simulink model "StandaloneDAQv07_R2014a"  (R2014a)
settings: Solver=FixedStepDiscrete  SolverMode=MultiTasking  StartTime=0.0  StopTime=inf  FixedStep=0.0005  RelTol=1e-3
values from neighbouring files (symbols this model uses):
  ANOMALY_INIT = 10    [DAQParams3_1ms_DDA.m]
  Calibration = getCalibrationParams_ATRIAS()    [DAQParams3_1ms_DDA.m]
  EnableFT = 0    [DAQParams3_1ms_DDA.m]
  EncoderAngleLimits = [60 240; 120 300; 60 240; 120 300; 60 240; 120 300; 60 240; 120 300; -30 30; -30 30; -inf inf; -inf inf; -inf inf; -inf inf; -30 30; -30 30; -inf inf; -90 90; -90 90]*pi/180    [DAQParams3_1ms_DDA.m]
  EncoderFiltSys = getDerivFilter(2, 5, 5, Ts)    [DAQParams3_1ms_DDA.m]
  EncoderThreshold = [5; 5; 5; 5; 5; 5; 5; 5; 5; 5; 250; 250; 250; 250; 5; 5; 5; 5; 5]*pi/180    [DAQParams3_1ms_DDA.m]
  IMUAngleLimits = [-180 180; -90 90; -90 90]*pi/180    [DAQParams3_1ms_DDA.m]
  IMUCommand = 70    [DAQParams3_1ms_DDA.m]
  IMUThreshold = 5*pi/180    (= 0.0872664625997)    [DAQParams3_1ms_DDA.m]
  MAX_ANOMALY = 30    [DAQParams3_1ms_DDA.m]
  MedullaCommand = 0    [DAQParams3_1ms_DDA.m]
  MicrostrainFiltSys = getDerivFilter(2, 5, 5, TsMicrostrain)    [DAQParams3_1ms_DDA.m]
  MODBUS_TIMEOUT = 0.02    [DAQParams3_1ms_DDA.m]
  ResetDAQ = 0    [DAQParams3_1ms_DDA.m]
  ResetYaw = 0    [DAQParams3_1ms_DDA.m]
  STREAMING_TIMEOUT = 0.1    [DAQParams3_1ms_DDA.m]
  TareFT = 0    [DAQParams3_1ms_DDA.m]
  Ts = 0.001    [DAQParams3_1ms_DDA.m]
  UseMicrostrainRate = 0    [DAQParams3_1ms_DDA.m]
undefined symbols (not defined in the file or in its folder): FTCalibration, GearOffset, IMUTorsoOffset, m_XR17D15x, standard
libraries: xpcethercatlib x167, speedgoatlib x13, dspswit3 x2, simulink x2, xpcseriallib x1, SpeedgoatModified x1
(part 1 of 4)
settings Model: xpc_rtwmakecfg_data=_xpcethercatlib_  ParamWorkspaceSource=ReferencedWorkspace  TunableVars=EnableFT,GearOffset,IMUCommand,IMUTorsoOffset,MedullaCommand,ResetDAQ,ResetYaw,TareFT  TunableVarsStorageClass=Auto,Auto,Auto,Auto,Auto,Auto,Auto,Auto  TunableVarsTypeQualifier=,,,,,,,  ExplicitPartitioning=on  Creator=bgbuss  LastModifiedBy=bgbuss
settings SolverCC: EnableConcurrentExecution=on
settings DataIOCC: LimitDataPoints=off
settings OptimizationCC: InlineParams=on  ExpressionDepthLimit=2147483647
settings DebuggingCC: UniqueDataStoreMsg=error  StateNameClashWarn=warning
settings HardwareCC: ProdIntDivRoundTo=Zero  ProdEndianess=LittleEndian  ProdHWDeviceType=Generic->32-bit x86 compatible
settings SFSimCC: SimUserIncludeDirs=./DynamicModel/c
settings RTWCC: SystemTargetFile=slrt.tlc  TLCOptions=-axPCModelStackSizeKB=128 -axPCMaxOverloads=100  TemplateMakefile=slrt_default_tmf  Description=Simulink Real-Time  ProcessScript=slrt_make_rtw_hook  RTWUseSimCustomCode=on  CustomInclude=./DynamicModel/c  CodeExecutionProfiling=on  CodeProfilingSaveOptions=AllData  RTWCompilerOptimization=On
settings CodeAppCC: MATLABSourceComments=on
settings SimulinkRealTimeCC: GeneratePreprocessorConditionals=Disable all  EnableShiftOperators=on  RL32LogBufSizeModifier=100000000  xPCTaskExecutionProfile=on  xPCRL32EventNumber=250000  xPCisModelTimeout=off  xPCModelTimeoutSecs=20

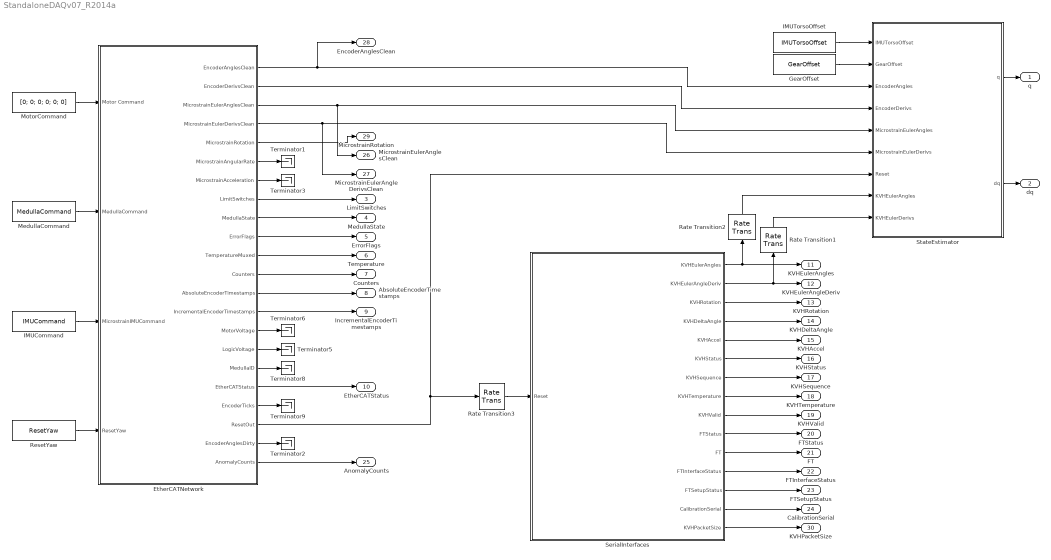
== system StandaloneDAQv07_R2014a ==
  EtherCATNetwork : Subsystem
  GearOffset : Constant  Value=GearOffset
  IMUCommand : Constant  Value=IMUCommand
  IMUTorsoOffset : Constant  Value=IMUTorsoOffset
  MedullaCommand : Constant  Value=MedullaCommand
  MotorCommand : Constant  Value=[0; 0; 0; 0; 0; 0]
  Rate Transition1 : RateTransition  OutPortSampleTime=Ts
  Rate Transition2 : RateTransition  OutPortSampleTime=Ts
  Rate Transition3 : RateTransition  OutPortSampleTime=0.001
  ResetYaw : Constant  Value=ResetYaw  OutDataTypeStr=boolean
  SerialInterfaces : Subsystem  TreatAsAtomicUnit=on  SystemSampleTime=0.001
  StateEstimator : Subsystem
  Terminator{1..3,5..6,8..9} (7 alike) : Terminator
  q : Outport
  dq : Outport  Port=2
  LimitSwitches : Outport  Port=3
  MedullaState : Outport  Port=4
  ErrorFlags : Outport  Port=5
  Temperature : Outport  Port=6
  Counters : Outport  Port=7
  AbsoluteEncoderTimestamps : Outport  Port=8
  IncrementalEncoderTimestamps : Outport  Port=9
  EtherCATStatus : Outport  Port=10
  KVHEulerAngles : Outport  Port=11
  KVHEulerAngleDeriv : Outport  Port=12
  KVHRotation : Outport  Port=13
  KVHDeltaAngle : Outport  Port=14
  KVHAccel : Outport  Port=15
  KVHStatus : Outport  Port=16
  KVHSequence : Outport  Port=17
  KVHTemperature : Outport  Port=18
  KVHValid : Outport  Port=19
  FTStatus : Outport  Port=20
  FT : Outport  Port=21
  FTInterfaceStatus : Outport  Port=22
  FTSetupStatus : Outport  Port=23
  CalibrationSerial : Outport  Port=24
  AnomalyCounts : Outport  Port=25
  MicrostrainEulerAnglesClean : Outport  Port=26
  MicrostrainEulerAngleDerivsClean : Outport  Port=27
  EncoderAnglesClean : Outport  Port=28
  MicrostrainRotation : Outport  Port=29
  KVHPacketSize : Outport  Port=30
  wires:
  EtherCATNetwork/8(LimitSwitches) -> LimitSwitches/1
  EtherCATNetwork/10(ErrorFlags) -> ErrorFlags/1
  EtherCATNetwork/15(MotorVoltage) -> Terminator6/1
  EtherCATNetwork/5(MicrostrainRotation) -> MicrostrainRotation/1
  EtherCATNetwork/9(MedullaState) -> MedullaState/1
  EtherCATNetwork/16(LogicVoltage) -> Terminator5/1
  EtherCATNetwork/11(TemperatureMuxed) -> Temperature/1
  EtherCATNetwork/18(EtherCATStatus) -> EtherCATStatus/1
  EtherCATNetwork/12(Counters) -> Counters/1
  StateEstimator/1(q) -> q/1
  StateEstimator/2(dq) -> dq/1
  EtherCATNetwork/22(AnomalyCounts) -> AnomalyCounts/1
  MotorCommand/1 -> EtherCATNetwork/1(Motor Command)
  MedullaCommand/1 -> EtherCATNetwork/2(MedullaCommand)
  IMUCommand/1 -> EtherCATNetwork/3(MicrostrainIMUCommand)
  EtherCATNetwork/17(MedullaID) -> Terminator8/1
  EtherCATNetwork/19(EncoderTicks) -> Terminator9/1
  EtherCATNetwork/7(MicrostrainAcceleration) -> Terminator3/1
  EtherCATNetwork/13(AbsoluteEncoderTimestamps) -> AbsoluteEncoderTimestamps/1
  EtherCATNetwork/14(IncrementalEncoderTimestamps) -> IncrementalEncoderTimestamps/1
  SerialInterfaces/10(FTStatus) -> FTStatus/1
  SerialInterfaces/11(FT) -> FT/1
  SerialInterfaces/12(FTInterfaceStatus) -> FTInterfaceStatus/1
  SerialInterfaces/13(FTSetupStatus) -> FTSetupStatus/1
  SerialInterfaces/14(CalibrationSerial) -> CalibrationSerial/1
  SerialInterfaces/3(KVHRotation) -> KVHRotation/1
  SerialInterfaces/2(KVHEulerAngleDeriv) -> KVHEulerAngleDeriv/1, Rate Transition1/1
  SerialInterfaces/1(KVHEulerAngles) -> Rate Transition2/1, KVHEulerAngles/1
  SerialInterfaces/7(KVHSequence) -> KVHSequence/1
  SerialInterfaces/8(KVHTemperature) -> KVHTemperature/1
  SerialInterfaces/5(KVHAccel) -> KVHAccel/1
  SerialInterfaces/9(KVHValid) -> KVHValid/1
  SerialInterfaces/6(KVHStatus) -> KVHStatus/1
  SerialInterfaces/4(KVHDeltaAngle) -> KVHDeltaAngle/1
  IMUTorsoOffset/1 -> StateEstimator/1(IMUTorsoOffset)
  GearOffset/1 -> StateEstimator/2(GearOffset)
  Rate Transition2/1 -> StateEstimator/8(KVHEulerAngles)
  EtherCATNetwork/20(ResetOut) -> StateEstimator/7(Reset), Rate Transition3/1
  EtherCATNetwork/1(EncoderAnglesClean) -> EncoderAnglesClean/1, StateEstimator/3(EncoderAngles)
  EtherCATNetwork/3(MicrostrainEulerAnglesClean) -> StateEstimator/5(MicrostrainEulerAngles), MicrostrainEulerAnglesClean/1
  EtherCATNetwork/4(MicrostrainEulerDerivsClean) -> StateEstimator/6(" MicrostrainEulerDerivs"), MicrostrainEulerAngleDerivsClean/1
  Rate Transition3/1 -> SerialInterfaces/1(Reset)
  EtherCATNetwork/2(EncoderDerivsClean) -> StateEstimator/4(EncoderDerivs)
  Rate Transition1/1 -> StateEstimator/9(KVHEulerDerivs)
  EtherCATNetwork/6(MicrostrainAngularRate) -> Terminator1/1
  EtherCATNetwork/21(EncoderAnglesDirty) -> Terminator2/1
  ResetYaw/1 -> EtherCATNetwork/4(ResetYaw)
  SerialInterfaces/15(KVHPacketSize) -> KVHPacketSize/1

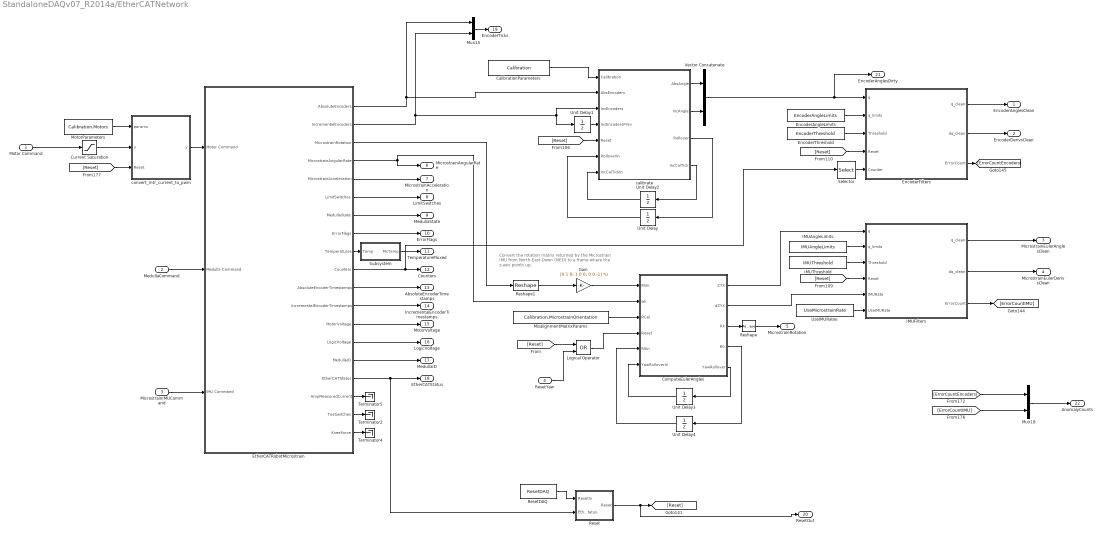
== system StandaloneDAQv07_R2014a/EtherCATNetwork ==
  note: Convert the rotation matrix returned by the
      | Microstrain IMU from North-East-Down
      | (NED) to a frame where the z-axis points up.
  Motor Command : Inport
  MedullaCommand : Inport  Port=2
  MicrostrainIMUCommand : Inport  Port=3
  ResetYaw : Inport  Port=4
  CalibrationParameters : Constant  Value=Calibration  OutDataTypeStr=Bus: RobotCalibrationBus
  ComputeEulerAngles : MATLAB Function  TreatAsAtomicUnit=on
  Current Saturation : Saturate  UpperLimit=50  LowerLimit=-50
  EncoderAngleLimits : Constant  Value=EncoderAngleLimits
  EncoderFilters : Subsystem  TreatAsAtomicUnit=on
  EncoderThreshold : Constant  Value=EncoderThreshold
  EtherCATRobotMicrostrain : Subsystem
  Gain : Gain  Gain=[0 1 0; 1 0 0; 0 0 -1]  Multiplication=Matrix(K*u)
  IMUAngleLimits : Constant  Value=IMUAngleLimits
  IMUFilters : Subsystem  TreatAsAtomicUnit=on
  IMUThreshold : Constant  Value=IMUThreshold
  Logical Operator : Logic  Operator=OR  OutDataTypeStr=boolean
  MisalignmentMatrixParams : Constant  Value=Calibration.MicrostrainOrientation
  MotorParameters : Constant  Value=Calibration.Motors
  Mux15 : Mux  Inputs=2
  Mux18 : Mux  Inputs=2
  Reset : Subsystem
  ResetDAQ : Constant  Value=ResetDAQ  OutDataTypeStr=boolean
  Reshape : Reshape
  Reshape1 : Reshape  OutputDimensionality=Customize  OutputDimensions=[3,3]
  Selector : Selector  IndexMode=Zero-based  InputPortWidth=7  Indices=[0 1 3 4 0 1 3 4 2 5 0 1 3 4 2 5 6 6 6]
  Subsystem : Subsystem
  Terminator2 : Terminator
  Terminator4 : Terminator
  Terminator5 : Terminator
  Unit Delay : UnitDelay  InitialCondition=zeros(9,1)  SampleTime=-1
  Unit Delay1 : UnitDelay  SampleTime=-1
  Unit Delay2 : UnitDelay  InitialCondition=zeros(6,1)  SampleTime=-1
  Unit Delay3 : UnitDelay  InitialCondition=[0; 0]  SampleTime=-1
  Unit Delay4 : UnitDelay  InitialCondition=zeros(3,3)  SampleTime=-1
  UseIMURates : Constant  Value=UseMicrostrainRate
  Vector Concatenate : Concatenate
  calibrate : MATLAB Function  TreatAsAtomicUnit=on
  convert_mtr_current_to_pwm : MATLAB Function  TreatAsAtomicUnit=on
  EncoderAnglesClean : Outport
  EncoderDerivsClean : Outport  Port=2
  MicrostrainEulerAnglesClean : Outport  Port=3
  MicrostrainEulerDerivsClean : Outport  Port=4
  MicrostrainRotation : Outport  Port=5
  MicrostrainAngularRate : Outport  Port=6
  MicrostrainAcceleration : Outport  Port=7
  LimitSwitches : Outport  Port=8
  MedullaState : Outport  Port=9
  ErrorFlags : Outport  Port=10
  TemperatureMuxed : Outport  Port=11
  Counters : Outport  Port=12
  AbsoluteEncoderTimestamps : Outport  Port=13
  IncrementalEncoderTimestamps : Outport  Port=14
  MotorVoltage : Outport  Port=15
  LogicVoltage : Outport  Port=16
  MedullaID : Outport  Port=17
  EtherCATStatus : Outport  Port=18
  EncoderTicks : Outport  Port=19
  ResetOut : Outport  Port=20
  EncoderAnglesDirty : Outport  Port=21
  AnomalyCounts : Outport  Port=22
  wires:
  EtherCATRobotMicrostrain/18(ToeSwitches) -> Terminator2/1
  EtherCATRobotMicrostrain/17(AmpMeasuredCurrent) -> Terminator5/1
  MicrostrainIMUCommand/1 -> EtherCATRobotMicrostrain/3(IMU Command)
  MedullaCommand/1 -> EtherCATRobotMicrostrain/2(Medulla Command)
  EtherCATRobotMicrostrain/16(EtherCATStatus) -> EtherCATStatus/1, Reset/2(EtherCATStatus)
  CalibrationParameters/1 -> calibrate/1(Calibration)
  calibrate/3(Rollover) -> Unit Delay/1
  Unit Delay/1 -> calibrate/6(RolloverIn)
  [Reset] -> calibrate/5(Reset)
  Reset/1(Reset) -> ResetOut/1, [Reset]
  ResetDAQ/1 -> Reset/1(ResetIn)
  Unit Delay1/1 -> calibrate/4(IncEncodersPrev)
  Unit Delay2/1 -> calibrate/7(IncCalTickIn)
  calibrate/4(IncCalTick) -> Unit Delay2/1
  [Reset] -> convert_mtr_current_to_pwm/3(Reset)
  Motor Command/1 -> Current Saturation/1
  MotorParameters/1 -> convert_mtr_current_to_pwm/1(params)
  Current Saturation/1 -> convert_mtr_current_to_pwm/2(u)
  convert_mtr_current_to_pwm/1(y) -> EtherCATRobotMicrostrain/1(Motor Command)
  Mux15/1 -> EncoderTicks/1
  EtherCATRobotMicrostrain/19(KneeForce) -> Terminator4/1
  EtherCATRobotMicrostrain/7(MedullaState) -> MedullaState/1
  Subsystem/1(MxTemp) -> TemperatureMuxed/1
  EtherCATRobotMicrostrain/9(Temperatures) -> Subsystem/1(Temp)
  EtherCATRobotMicrostrain/8(ErrorFlags) -> ErrorFlags/1
  EtherCATRobotMicrostrain/6(LimitSwitches) -> LimitSwitches/1
  EtherCATRobotMicrostrain/13(MotorVoltage) -> MotorVoltage/1
  EtherCATRobotMicrostrain/14(LogicVoltage) -> LogicVoltage/1
  EtherCATRobotMicrostrain/5(MicrostrainAcceleration) -> MicrostrainAcceleration/1
  EtherCATRobotMicrostrain/11(AbsoluteEncoderTimestamps) -> AbsoluteEncoderTimestamps/1
  EtherCATRobotMicrostrain/12(IncrementalEncoderTimestamps) -> IncrementalEncoderTimestamps/1
  EtherCATRobotMicrostrain/15(MedullaID) -> MedullaID/1
  EtherCATRobotMicrostrain/1(AbsoluteEncoders) -> Mux15/1, calibrate/2(AbsEncoders)
  EtherCATRobotMicrostrain/2(IncrementalEncoders) -> Mux15/2, calibrate/3(IncEncoders), Unit Delay1/1
  ComputeEulerAngles/1(ZYX) -> IMUFilters/1(q)
  [Reset] -> IMUFilters/4(Reset)
  IMUFilters/3(ErrorCount) -> [ErrorCountIMU]
  IMUThreshold/1 -> IMUFilters/3(Threshold)
  EtherCATRobotMicrostrain/10(Counters) -> Selector/1, Counters/1
  IMUAngleLimits/1 -> IMUFilters/2(q_limits)
  Selector/1 -> EncoderFilters/5(Counter)
  UseIMURates/1 -> IMUFilters/6(UseIMURate)
  EncoderFilters/3(ErrorCount) -> [ErrorCountEncoders]
  IMUFilters/2(dq_clean) -> MicrostrainEulerDerivsClean/1
  [Reset] -> EncoderFilters/4(Reset)
  EncoderAngleLimits/1 -> EncoderFilters/2(q_limits)
  EncoderFilters/1(q_clean) -> EncoderAnglesClean/1
  IMUFilters/1(q_clean) -> MicrostrainEulerAnglesClean/1
  EncoderFilters/2(dq_clean) -> EncoderDerivsClean/1
  EncoderThreshold/1 -> EncoderFilters/3(Threshold)
  calibrate/1(AbsAngle) -> Vector Concatenate/1
  calibrate/2(IncAngle) -> Vector Concatenate/2
  Vector Concatenate/1 -> EncoderAnglesDirty/1, EncoderFilters/1(q)
  ComputeEulerAngles/2(dZYX) -> IMUFilters/5(IMURate)
  Mux18/1 -> AnomalyCounts/1
  [ErrorCountEncoders] -> Mux18/1
  [ErrorCountIMU] -> Mux18/2
  MisalignmentMatrixParams/1 -> ComputeEulerAngles/3(RCal)
  Unit Delay4/1 -> ComputeEulerAngles/5(R0In)
  ComputeEulerAngles/4(R0) -> Unit Delay4/1
  ComputeEulerAngles/3(Rk) -> Reshape/1
  [Reset] -> Logical Operator/1
  Reshape/1 -> MicrostrainRotation/1
  EtherCATRobotMicrostrain/3(MicrostrainRotation) -> Reshape1/1
  EtherCATRobotMicrostrain/4(MicrostrainAngularRate) -> ComputeEulerAngles/2(wk), MicrostrainAngularRate/1
  ComputeEulerAngles/5(YawRollover) -> Unit Delay3/1
  Unit Delay3/1 -> ComputeEulerAngles/6(YawRolloverIn)
  ResetYaw/1 -> Logical Operator/2
  Logical Operator/1 -> ComputeEulerAngles/4(Reset)
  Reshape1/1 -> Gain/1
  Gain/1 -> ComputeEulerAngles/1(RkIn)

== system StandaloneDAQv07_R2014a/SerialInterfaces ==
  Reset : Inport
  EnableFT : Constant  Value=EnableFT  OutDataTypeStr=boolean
  FTInterface : Subsystem
  KVH : Subsystem
  ResetYaw : Constant  Value=ResetYaw  OutDataTypeStr=boolean
  TareFT : Constant  Value=TareFT  OutDataTypeStr=boolean
  KVHEulerAngles : Outport
  KVHEulerAngleDeriv : Outport  Port=2
  KVHRotation : Outport  Port=3
  KVHDeltaAngle : Outport  Port=4
  KVHAccel : Outport  Port=5
  KVHStatus : Outport  Port=6
  KVHSequence : Outport  Port=7
  KVHTemperature : Outport  Port=8
  KVHValid : Outport  Port=9
  FTStatus : Outport  Port=10
  FT : Outport  Port=11
  FTInterfaceStatus : Outport  Port=12
  FTSetupStatus : Outport  Port=13
  CalibrationSerial : Outport  Port=14
  KVHPacketSize : Outport  Port=15
  wires:
  KVH/4(DeltaAngle) -> KVHDeltaAngle/1
  KVH/5(Accel) -> KVHAccel/1
  KVH/7(Sequence) -> KVHSequence/1
  KVH/6(Status) -> KVHStatus/1
  KVH/8(Temperature) -> KVHTemperature/1
  KVH/9(Valid) -> KVHValid/1
  ResetYaw/1 -> KVH/1(ResetYaw)
  KVH/1(EulerAngles) -> KVHEulerAngles/1
  KVH/2(EulerAngleDerivatives) -> KVHEulerAngleDeriv/1
  FTInterface/4(FTSetupStatus) -> FTSetupStatus/1
  FTInterface/1(FTStatus) -> FTStatus/1
  FTInterface/5(CalibrationSerial) -> CalibrationSerial/1
  FTInterface/3(FTInterfaceStatus) -> FTInterfaceStatus/1
  TareFT/1 -> FTInterface/1(Tare)
  Reset/1 -> FTInterface/2(Reset), KVH/2(Reset)
  FTInterface/2(FT) -> FT/1
  KVH/3(Rk) -> KVHRotation/1
  EnableFT/1 -> FTInterface/Enable
  KVH/10(PacketSize) -> KVHPacketSize/1

== system StandaloneDAQv07_R2014a/StateEstimator ==
  IMUTorsoOffset : Inport
  GearOffset : Inport  Port=2
  EncoderAngles : Inport  Port=3
  EncoderDerivs : Inport  Port=4
  MicrostrainEulerAngles : Inport  Port=5
  " MicrostrainEulerDerivs" : Inport  Port=6
  Reset : Inport  Port=7
  KVHEulerAngles : Inport  Port=8
  KVHEulerDerivs : Inport  Port=9
  GeneralizedCoordinates : MATLAB Function  TreatAsAtomicUnit=on
  Switch : Switch  Criteria=u2 > Threshold
  Switch1 : Switch  Criteria=u2 > Threshold
  UseIMU : Constant
  UseKVH : Constant
  UseMotorIncEncoders : Constant
  q : Outport
  dq : Outport  Port=2
  wires:
  UseIMU/1 -> GeneralizedCoordinates/6(UseIMU)
  GearOffset/1 -> GeneralizedCoordinates/8(GearOffset)
  UseMotorIncEncoders/1 -> GeneralizedCoordinates/5(UseMotorIncEncoders)
  IMUTorsoOffset/1 -> GeneralizedCoordinates/7(IMUTorsoOffset)
  GeneralizedCoordinates/2(dq_clean) -> dq/1
  GeneralizedCoordinates/1(q_clean) -> q/1
  Reset/1 -> GeneralizedCoordinates/9(Reset)
  EncoderAngles/1 -> GeneralizedCoordinates/1(EncoderAngles)
  EncoderDerivs/1 -> GeneralizedCoordinates/2(EncoderVelocities)
  KVHEulerAngles/1 -> Switch/1
  MicrostrainEulerAngles/1 -> Switch/3
  Switch/1 -> GeneralizedCoordinates/3(IMUAngles)
  UseKVH/1 -> Switch1/2, Switch/2
  KVHEulerDerivs/1 -> Switch1/1
  " MicrostrainEulerDerivs"/1 -> Switch1/3
  Switch1/1 -> GeneralizedCoordinates/4(IMUVelocities)

== system StandaloneDAQv07_R2014a/EtherCATNetwork/EncoderFilters ==
  q : Inport  Partition=on  PartitionDimension=1  PartitionWidth=1
  q_limits : Inport  Port=2  Partition=on  PartitionDimension=1  PartitionWidth=1
  Threshold : Inport  Port=3  Partition=on  PartitionDimension=1  PartitionWidth=1
  Reset : Inport  Port=4  Partition=off
  Counter : Inport  Port=5  Partition=on  PartitionDimension=1  PartitionWidth=1
  CheckAndFilterEncoder : Subsystem
  For Each : ForEach  DisableCoverage=on  IndexMode=One-based
  q_clean : Outport  ConcatenationDimension=1
  dq_clean : Outport  Port=2  ConcatenationDimension=1
  ErrorCount : Outport  Port=3  ConcatenationDimension=1
  wires:
  Counter/1 -> CheckAndFilterEncoder/5(Counter)
  Reset/1 -> CheckAndFilterEncoder/4(Reset)
  CheckAndFilterEncoder/2(dq_clean) -> dq_clean/1
  q_limits/1 -> CheckAndFilterEncoder/2(q_limits)
  CheckAndFilterEncoder/3(ErrorCount) -> ErrorCount/1
  CheckAndFilterEncoder/1(q_clean) -> q_clean/1
  Threshold/1 -> CheckAndFilterEncoder/3(Threshold)
  q/1 -> CheckAndFilterEncoder/1(q_daq)

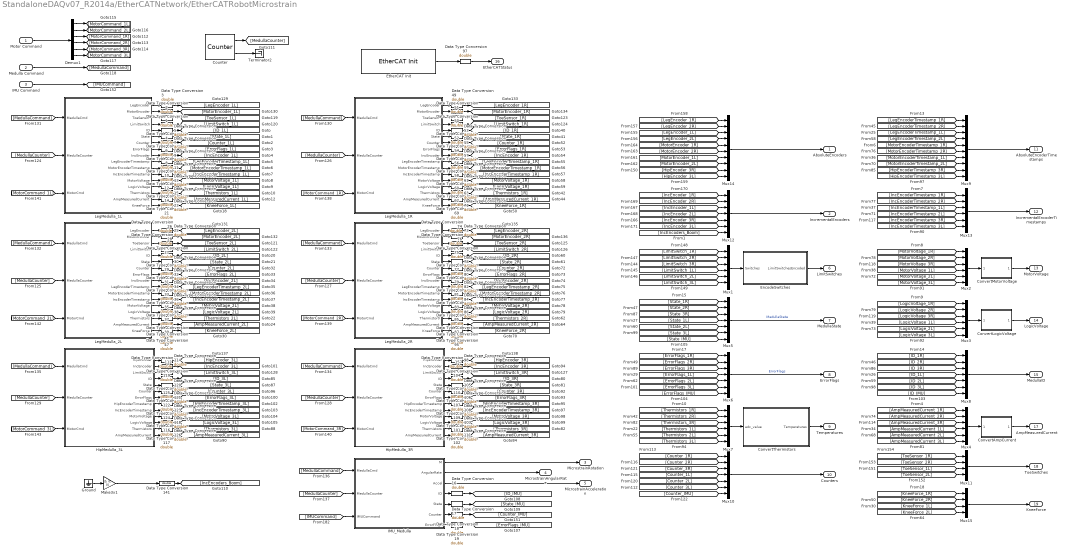
== system StandaloneDAQv07_R2014a/EtherCATNetwork/EtherCATRobotMicrostrain ==
  Motor Command : Inport
  Medulla Command : Inport  Port=2
  IMU Command : Inport  Port=3
  ConvertAmpCurrent : MATLAB Function  TreatAsAtomicUnit=on
  ConvertLogicVoltage : MATLAB Function  TreatAsAtomicUnit=on
  ConvertMotorVoltage : MATLAB Function  TreatAsAtomicUnit=on
  ConvertThermistors : MATLAB Function  TreatAsAtomicUnit=on
  Counter : dspswit3/Counter  Direction=Up  CountEvent=Free running  CounterSize=User defined  MaxCount=65535  InitialCount=0  Output=Count and Hit  HitValue=32  ResetInput=off  SamplesPerFrame=1  Ts=Ts  CntDtype=double  HitDtype=Logical
  Data Type Conversion{1..19,21,23,25..39,45,47,49..63,69,71,73..87,93,95,97..98,101..112,114,116..126,141,157} (100 alike) : DataTypeConversion  OutDataTypeStr=double
  Demux1 : Demux  Outputs=6
  EncodeSwitches : MATLAB Function  TreatAsAtomicUnit=on
  EtherCAT Init : xpcethercatlib/EtherCAT Init   Priority=0  config_file='FullWithMicrostrain-SlaveMode-500us-eni.xml'  device_id=0  pci_bus=10  pci_slot=0  enaDebug=off  enaDC=on  errLink=off  masterDbg=off  stateChgDbg=off  baseClock=off  masterCfg=off  logFile='c:\dbglog.txt'  sample_time=0.000500
  Ground : Ground
  HipMedulla_3L : Subsystem
  HipMedulla_3R : Subsystem
  IMU_Medulla : Subsystem
  LegMedulla_1L : Subsystem
  LegMedulla_1R : Subsystem
  LegMedulla_2L : Subsystem
  LegMedulla_2R : Subsystem
  Make3x1 : Gain  Gain=[0; 0; 0]
  Mux{1..4,7,13} (6 alike) : Mux  Inputs=6
  Mux{5..6,8,10,12} (5 alike) : Mux  Inputs=7
  Mux11 : Mux
  Mux14 : Mux  Inputs=10
  Mux15 : Mux
  Mux9 : Mux  Inputs=10
  Terminator2 : Terminator
  AbsoluteEncoders : Outport
  IncrementalEncoders : Outport  Port=2
  MicrostrainRotation : Outport  Port=3
  MicrostrainAngularRate : Outport  Port=4
  MicrostrainAcceleration : Outport  Port=5
  LimitSwitches : Outport  Port=6
  MedullaState : Outport  Port=7
  ErrorFlags : Outport  Port=8
  Temperatures : Outport  Port=9
  Counters : Outport  Port=10
  AbsoluteEncoderTimestamps : Outport  Port=11
  IncrementalEncoderTimestamps : Outport  Port=12
  MotorVoltage : Outport  Port=13
  LogicVoltage : Outport  Port=14
  MedullaID : Outport  Port=15
  EtherCATStatus : Outport  Port=16
  AmpMeasuredCurrent : Outport  Port=17
  ToeSwitches : Outport  Port=18
  KneeForce : Outport  Port=19
  wires:
  Data Type Conversion97/1 -> EtherCATStatus/1
  EtherCAT Init/1 -> Data Type Conversion97/1
  Mux11/1 -> ToeSwitches/1
  EncodeSwitches/1(LimitSwitchesEncoded) -> LimitSwitches/1
  LegMedulla_1L/2(MotorEncoder) -> Data Type Conversion1/1
  LegMedulla_1L/3(ToeSensor) -> Data Type Conversion2/1
  LegMedulla_1L/4(LimitSwitch) -> Data Type Conversion4/1
  LegMedulla_1L/5(ID) -> Data Type Conversion5/1
  LegMedulla_1L/6(State) -> Data Type Conversion6/1
  LegMedulla_1L/7(Counter) -> Data Type Conversion7/1
  LegMedulla_1L/8(ErrorFlags) -> Data Type Conversion8/1
  LegMedulla_1L/9(IncEncoder) -> Data Type Conversion9/1
  LegMedulla_1L/10(LegEncoderTimestamp) -> Data Type Conversion10/1
  LegMedulla_1L/11(MotorEncoderTimestamp) -> Data Type Conversion11/1
  LegMedulla_1L/12(IncEncoderTimestamp) -> Data Type Conversion12/1
  LegMedulla_1L/13(MotorVoltage) -> Data Type Conversion13/1
  LegMedulla_1L/14(LogicVoltage) -> Data Type Conversion14/1
  LegMedulla_1L/15(Thermistors) -> Data Type Conversion15/1
  LegMedulla_1L/16(AmpMeasuredCurrent) -> Data Type Conversion21/1
  LegMedulla_1L/17(KneeForce) -> Data Type Conversion23/1
  LegMedulla_2L/1(LegEncoder) -> Data Type Conversion25/1
  LegMedulla_2L/2(MotorEncoder) -> Data Type Conversion26/1
  LegMedulla_2L/3(ToeSensor) -> Data Type Conversion27/1
  LegMedulla_2L/4(LimitSwitch) -> Data Type Conversion28/1
  LegMedulla_2L/5(ID) -> Data Type Conversion29/1
  LegMedulla_2L/6(State) -> Data Type Conversion30/1
  LegMedulla_2L/7(Counter) -> Data Type Conversion31/1
  LegMedulla_2L/8(ErrorFlags) -> Data Type Conversion32/1
  LegMedulla_2L/9(IncEncoder) -> Data Type Conversion33/1
  LegMedulla_2L/10(LegEncoderTimestamp) -> Data Type Conversion34/1
  LegMedulla_2L/11(MotorEncoderTimestamp) -> Data Type Conversion35/1
  LegMedulla_2L/12(IncEncoderTimestamp) -> Data Type Conversion36/1
  LegMedulla_2L/13(MotorVoltage) -> Data Type Conversion37/1
  LegMedulla_2L/14(LogicVoltage) -> Data Type Conversion38/1
  LegMedulla_2L/15(Thermistors) -> Data Type Conversion39/1
  LegMedulla_2L/16(AmpMeasuredCurrent) -> Data Type Conversion45/1
  LegMedulla_2L/17(KneeForce) -> Data Type Conversion47/1
  LegMedulla_1R/3(ToeSensor) -> Data Type Conversion51/1
  LegMedulla_1R/4(LimitSwitch) -> Data Type Conversion52/1
  LegMedulla_1R/5(ID) -> Data Type Conversion53/1
  LegMedulla_1R/6(State) -> Data Type Conversion54/1
  LegMedulla_1R/7(Counter) -> Data Type Conversion55/1
  LegMedulla_1R/8(ErrorFlags) -> Data Type Conversion56/1
  LegMedulla_1R/9(IncEncoder) -> Data Type Conversion57/1
  LegMedulla_1R/10(LegEncoderTimestamp) -> Data Type Conversion58/1
  LegMedulla_1R/11(MotorEncoderTimestamp) -> Data Type Conversion59/1
  LegMedulla_1R/12(IncEncoderTimestamp) -> Data Type Conversion60/1
  LegMedulla_1R/13(MotorVoltage) -> Data Type Conversion61/1
  LegMedulla_1R/14(LogicVoltage) -> Data Type Conversion62/1
  LegMedulla_1R/15(Thermistors) -> Data Type Conversion63/1
  LegMedulla_1R/16(AmpMeasuredCurrent) -> Data Type Conversion69/1
  LegMedulla_1R/17(KneeForce) -> Data Type Conversion71/1
  LegMedulla_2R/4(LimitSwitch) -> Data Type Conversion76/1
  LegMedulla_2R/5(ID) -> Data Type Conversion77/1
  LegMedulla_2R/6(State) -> Data Type Conversion78/1
  LegMedulla_2R/7(Counter) -> Data Type Conversion79/1
  LegMedulla_2R/8(ErrorFlags) -> Data Type Conversion80/1
  LegMedulla_2R/9(IncEncoder) -> Data Type Conversion81/1
  LegMedulla_2R/10(LegEncoderTimestamp) -> Data Type Conversion82/1
  LegMedulla_2R/11(MotorEncoderTimestamp) -> Data Type Conversion83/1
  LegMedulla_2R/12(IncEncoderTimestamp) -> Data Type Conversion84/1
  LegMedulla_2R/13(MotorVoltage) -> Data Type Conversion85/1
  LegMedulla_2R/14(LogicVoltage) -> Data Type Conversion86/1
  LegMedulla_2R/15(Thermistor0) -> Data Type Conversion87/1
  LegMedulla_2R/16(AmpMeasuredCurrent) -> Data Type Conversion93/1
  LegMedulla_2R/17(KneeForce) -> Data Type Conversion95/1
  Medulla Command/1 -> [MedullaCommand]
  Counter/2 -> Terminator2/1
  LegMedulla_2R/1(LegEncoder) -> Data Type Conversion73/1
  LegMedulla_2R/2(MotorEncoder) -> Data Type Conversion74/1
  LegMedulla_2R/3(ToeSensor) -> Data Type Conversion75/1
  Data Type Conversion53/1 -> [ID_1R]
  Data Type Conversion54/1 -> [State_1R]
  Data Type Conversion55/1 -> [Counter_1R]
  Data Type Conversion56/1 -> [ErrorFlags_1R]
  Data Type Conversion57/1 -> [IncEncoder_1R]
  Data Type Conversion58/1 -> [LegEncoderTimestamp_1R]
  Data Type Conversion59/1 -> [MotorEncoderTimestamp_1R]
  Data Type Conversion60/1 -> [IncEncoderTimestamp_1R]
  Data Type Conversion61/1 -> [MotorVoltage_1R]
  Data Type Conversion62/1 -> [LogicVoltage_1R]
  Data Type Conversion63/1 -> [Thermistors_1R]
  Data Type Conversion69/1 -> [AmpMeasuredCurrent_1R]
  Data Type Conversion71/1 -> [KneeForce_1R]
  Data Type Conversion77/1 -> [ID_2R]
  Data Type Conversion78/1 -> [State_2R]
  Data Type Conversion79/1 -> [Counter_2R]
  Data Type Conversion80/1 -> [ErrorFlags_2R]
  Data Type Conversion81/1 -> [IncEncoder_2R]
  Data Type Conversion82/1 -> [LegEncoderTimestamp_2R]
  Data Type Conversion83/1 -> [MotorEncoderTimestamp_2R]
  Data Type Conversion84/1 -> [IncEncoderTimestamp_2R]
  Data Type Conversion85/1 -> [MotorVoltage_2R]
  Data Type Conversion86/1 -> [LogicVoltage_2R]
  Data Type Conversion87/1 -> [Thermistors_2R]
  Data Type Conversion93/1 -> [AmpMeasuredCurrent_2R]
  Data Type Conversion95/1 -> [KneeForce_2R]
  Data Type Conversion111/1 -> [AmpMeasuredCurrent_3R]
  LegMedulla_1R/2(MotorEncoder) -> Data Type Conversion50/1
  LegMedulla_1L/1(LegEncoder) -> Data Type Conversion3/1
  LegMedulla_1R/1(LegEncoder) -> Data Type Conversion49/1
  Data Type Conversion5/1 -> [ID_1L]
  Data Type Conversion6/1 -> [State_1L]
  Data Type Conversion7/1 -> [Counter_1L]
  Data Type Conversion29/1 -> [ID_2L]
  Data Type Conversion30/1 -> [State_2L]
  Data Type Conversion31/1 -> [Counter_2L]
  Data Type Conversion32/1 -> [ErrorFlags_2L]
  Data Type Conversion33/1 -> [IncEncoder_2L]
  Data Type Conversion34/1 -> [LegEncoderTimestamp_2L]
  Data Type Conversion35/1 -> [MotorEncoderTimestamp_2L]
  Data Type Conversion36/1 -> [IncEncoderTimestamp_2L]
  Data Type Conversion37/1 -> [MotorVoltage_2L]
  Data Type Conversion38/1 -> [LogicVoltage_2L]
  Data Type Conversion39/1 -> [Thermistors_2L]
  Data Type Conversion45/1 -> [AmpMeasuredCurrent_2L]
  Data Type Conversion47/1 -> [KneeForce_2L]
  Data Type Conversion102/1 -> [Thermistors_3R]
  Data Type Conversion103/1 -> [LogicVoltage_3R]
  Data Type Conversion101/1 -> [MotorVoltage_3R]
  Data Type Conversion108/1 -> [IncEncoderTimestamp_3R]
  Data Type Conversion109/1 -> [HipEncoderTimestamp_3R]
  Data Type Conversion104/1 -> [IncEncoder_3R]
  Data Type Conversion106/1 -> [ErrorFlags_3R]
  Data Type Conversion107/1 -> [Counter_3R]
  Data Type Conversion105/1 -> [State_3R]
  Data Type Conversion110/1 -> [ID_3R]
  Data Type Conversion98/1 -> [HipEncoder_3R]
  HipMedulla_3R/1(HipEncoder) -> Data Type Conversion98/1
  HipMedulla_3R/2(IncEncoder) -> Data Type Conversion104/1
  HipMedulla_3R/3(LimitSwitch) -> Data Type Conversion157/1
  HipMedulla_3R/4(ID) -> Data Type Conversion110/1
  HipMedulla_3R/5(State) -> Data Type Conversion105/1
  HipMedulla_3R/6(Counter) -> Data Type Conversion107/1
  HipMedulla_3R/7(ErrorFlags) -> Data Type Conversion106/1
  HipMedulla_3R/8(HipEncoderTimestamp) -> Data Type Conversion109/1
  HipMedulla_3R/9(IncEncoderTimestamp) -> Data Type Conversion108/1
  HipMedulla_3R/10(MotorVoltage) -> Data Type Conversion101/1
  HipMedulla_3R/11(LogicVoltage) -> Data Type Conversion103/1
  HipMedulla_3R/12(Thermistors) -> Data Type Conversion102/1
  HipMedulla_3R/13(AmpMeasuredCurrent) -> Data Type Conversion111/1
  HipMedulla_3L/3(LimitSwitch) -> Data Type Conversion112/1
  Data Type Conversion114/1 -> [HipEncoder_3L]
  HipMedulla_3L/1(HipEncoder) -> Data Type Conversion114/1
  HipMedulla_3L/2(IncEncoder) -> Data Type Conversion119/1
  Data Type Conversion126/1 -> [AmpMeasuredCurrent_3L]
  Data Type Conversion117/1 -> [Thermistors_3L]
  Data Type Conversion118/1 -> [LogicVoltage_3L]
  Data Type Conversion116/1 -> [MotorVoltage_3L]
  Data Type Conversion123/1 -> [IncEncoderTimestamp_3L]
  Data Type Conversion124/1 -> [HipEncoderTimestamp_3L]
  Data Type Conversion119/1 -> [IncEncoder_3L]
  Data Type Conversion121/1 -> [ErrorFlags_3L]
  Data Type Conversion122/1 -> [Counter_3L]
  Data Type Conversion120/1 -> [State_3L]
  Data Type Conversion125/1 -> [ID_3L]
  HipMedulla_3L/4(ID) -> Data Type Conversion125/1
  HipMedulla_3L/5(State) -> Data Type Conversion120/1
  HipMedulla_3L/6(Counter) -> Data Type Conversion122/1
  HipMedulla_3L/7(ErrorFlags) -> Data Type Conversion121/1
  HipMedulla_3L/8(HipEncoderTimestamp) -> Data Type Conversion124/1
  HipMedulla_3L/9(IncEncoderTimestamp) -> Data Type Conversion123/1
  HipMedulla_3L/10(MotorVoltage) -> Data Type Conversion116/1
  HipMedulla_3L/11(LogicVoltage) -> Data Type Conversion118/1
  HipMedulla_3L/12(Thermistors) -> Data Type Conversion117/1
  HipMedulla_3L/13(AmpMeasuredCurrent) -> Data Type Conversion126/1
  Mux1/1 -> EncodeSwitches/1(Switches)
  Data Type Conversion8/1 -> [ErrorFlags_1L]
  Data Type Conversion9/1 -> [IncEncoder_1L]
  Data Type Conversion10/1 -> [LegEncoderTimestamp_1L]
  Data Type Conversion11/1 -> [MotorEncoderTimestamp_1L]
  Data Type Conversion12/1 -> [IncEncoderTimestamp_1L]
  Data Type Conversion13/1 -> [MotorVoltage_1L]
  Data Type Conversion14/1 -> [LogicVoltage_1L]
  Data Type Conversion15/1 -> [Thermistors_1L]
  Data Type Conversion21/1 -> [AmpMeasuredCurrent_1L]
  Data Type Conversion23/1 -> [KneeForce_1L]
  [MotorVoltage_1R] -> Mux2/1
  [MotorVoltage_2R] -> Mux2/2
  [MotorVoltage_3R] -> Mux2/3
  [MotorVoltage_1L] -> Mux2/4
  [MotorVoltage_2L] -> Mux2/5
  [MotorVoltage_3L] -> Mux2/6
  [LogicVoltage_1R] -> Mux3/1
  [LogicVoltage_2R] -> Mux3/2
  [LogicVoltage_3R] -> Mux3/3
  [LogicVoltage_1L] -> Mux3/4
  [LogicVoltage_2L] -> Mux3/5
  [LogicVoltage_3L] -> Mux3/6
  [AmpMeasuredCurrent_1R] -> Mux4/1
  [AmpMeasuredCurrent_2R] -> Mux4/2
  [AmpMeasuredCurrent_3R] -> Mux4/3
  [AmpMeasuredCurrent_1L] -> Mux4/4
  [AmpMeasuredCurrent_2L] -> Mux4/5
  [AmpMeasuredCurrent_3L] -> Mux4/6
  [State_1R] -> Mux5/1
  [State_2R] -> Mux5/2
  [State_3R] -> Mux5/3
  [State_1L] -> Mux5/4
  [State_2L] -> Mux5/5
  [State_3L] -> Mux5/6
  [ErrorFlags_1R] -> Mux6/1
  [ErrorFlags_2R] -> Mux6/2
  [ErrorFlags_3R] -> Mux6/3
  [ErrorFlags_1L] -> Mux6/4
  [ErrorFlags_2L] -> Mux6/5
  [ErrorFlags_3L] -> Mux6/6
  [ErrorFlags_IMU] -> Mux6/7
  [State_IMU] -> Mux5/7
  Mux2/1 -> ConvertMotorVoltage/1(adc_value)
  Mux3/1 -> ConvertLogicVoltage/1(adc_value)
  Mux4/1 -> ConvertAmpCurrent/1(adc_value)
  ConvertMotorVoltage/1(motorVoltage) -> MotorVoltage/1
  ConvertLogicVoltage/1(logicVoltage) -> LogicVoltage/1
  ConvertAmpCurrent/1(measuredCurrent) -> AmpMeasuredCurrent/1
  Mux5/1 -> MedullaState/1  "MedullaState"
  Mux6/1 -> ErrorFlags/1  "ErrorFlags"
  Mux10/1 -> Counters/1
  [Counter_1R] -> Mux10/1
  [Counter_2R] -> Mux10/2
  [Counter_3R] -> Mux10/3
  [Counter_1L] -> Mux10/4
  [Counter_2L] -> Mux10/5
  [Counter_3L] -> Mux10/6
  [Counter_IMU] -> Mux10/7
  Counter/1 -> [MedullaCounter]
  [MedullaCounter] -> LegMedulla_1L/2(MedullaCounter)
  [MedullaCounter] -> HipMedulla_3L/2(MedullaCounter)
  [MedullaCounter] -> HipMedulla_3R/2(MedullaCounter)
  [MedullaCounter] -> LegMedulla_2R/2(MedullaCounter)
  [MedullaCounter] -> LegMedulla_1R/2(MedullaCounter)
  [MedullaCounter] -> LegMedulla_2L/2(MedullaCounter)
  [MedullaCommand] -> LegMedulla_1R/1(MedullaCmd)
  [MedullaCommand] -> LegMedulla_2R/1(MedullaCmd)
  [MedullaCommand] -> LegMedulla_2L/1(MedullaCmd)
  [MedullaCommand] -> LegMedulla_1L/1(MedullaCmd)
  [MedullaCommand] -> HipMedulla_3R/1(MedullaCmd)
  [MedullaCommand] -> HipMedulla_3L/1(MedullaCmd)
  [MotorCommand_1L] -> LegMedulla_1L/3(MotorCmd)
  [MotorCommand_2L] -> LegMedulla_2L/3(MotorCmd)
  [MotorCommand_1R] -> LegMedulla_1R/3(MotorCmd)
  [MotorCommand_2R] -> LegMedulla_2R/3(MotorCmd)
  [MotorCommand_3R] -> HipMedulla_3R/3(MotorCmd)
  Demux1/6 -> [MotorCommand_3L]
  [MotorCommand_3L] -> HipMedulla_3L/3(MotorCmd)
  Demux1/1 -> [MotorCommand_1L]
  Demux1/2 -> [MotorCommand_2L]
  Demux1/3 -> [MotorCommand_1R]
  Demux1/4 -> [MotorCommand_2R]
  Demux1/5 -> [MotorCommand_3R]
  Data Type Conversion157/1 -> [LimitSwitch_3R]
  Data Type Conversion112/1 -> [LimitSwitch_3L]
  [LimitSwitch_1R] -> Mux1/1
  [LimitSwitch_2R] -> Mux1/2
  [LimitSwitch_3R] -> Mux1/3
  [LimitSwitch_1L] -> Mux1/4
  [LimitSwitch_2L] -> Mux1/5
  [LimitSwitch_3L] -> Mux1/6
  [ToeSensor_1R] -> Mux11/1
  [ToeSensor_2R] -> Mux11/2
  [ToeSensor_1L] -> Mux11/3
  [ToeSensor_2L] -> Mux11/4
  Data Type Conversion76/1 -> [LimitSwitch_2R]
  Data Type Conversion75/1 -> [ToeSensor_2R]
  Data Type Conversion51/1 -> [ToeSensor_1R]
  Data Type Conversion52/1 -> [LimitSwitch_1R]
  Data Type Conversion27/1 -> [ToeSensor_2L]
  Data Type Conversion28/1 -> [LimitSwitch_2L]
  Data Type Conversion2/1 -> [ToeSensor_1L]
  Data Type Conversion4/1 -> [LimitSwitch_1L]
  Data Type Conversion3/1 -> [LegEncoder_1L]
  Data Type Conversion1/1 -> [MotorEncoder_1L]
  Data Type Conversion25/1 -> [LegEncoder_2L]
  Data Type Conversion26/1 -> [MotorEncoder_2L]
  Data Type Conversion49/1 -> [LegEncoder_1R]
  Data Type Conversion50/1 -> [MotorEncoder_1R]
  Data Type Conversion73/1 -> [LegEncoder_2R]
  Data Type Conversion74/1 -> [MotorEncoder_2R]
  [IncEncoder_1R] -> Mux12/1
  [IncEncoder_2R] -> Mux12/2
  [IncEncoder_3R] -> Mux12/5
  [IncEncoder_1L] -> Mux12/3
  [IncEncoder_2L] -> Mux12/4
  [IncEncoder_3L] -> Mux12/6
  [LegEncoder_1R] -> Mux14/1
  [LegEncoder_2R] -> Mux14/2
  [LegEncoder_1L] -> Mux14/3
  [LegEncoder_2L] -> Mux14/4
  IMU Command/1 -> [IMUCommand]
  [MotorEncoder_1R] -> Mux14/5
  [MotorEncoder_2R] -> Mux14/6
  [MotorEncoder_1L] -> Mux14/7
  [MotorEncoder_2L] -> Mux14/8
  [HipEncoder_3R] -> Mux14/9
  [HipEncoder_3L] -> Mux14/10
  [MedullaCommand] -> IMU_Medulla/1(MedullaCmd)
  [MedullaCounter] -> IMU_Medulla/2(MedullaCounter)
  [IMUCommand] -> IMU_Medulla/3(IMUCommand)
  IMU_Medulla/1(M) -> MicrostrainRotation/1
  IMU_Medulla/4(ID) -> Data Type Conversion16/1
  IMU_Medulla/5(State) -> Data Type Conversion17/1
  IMU_Medulla/6(Counter) -> Data Type Conversion18/1
  IMU_Medulla/7(ErrorFlags) -> Data Type Conversion19/1
  Mux7/1 -> ConvertThermistors/1(adc_value)
  ConvertThermistors/1(Temperatures) -> Temperatures/1
  Motor Command/1 -> Demux1/1
  [Thermistors_1R] -> Mux7/1
  [Thermistors_2L] -> Mux7/5
  [Thermistors_1L] -> Mux7/4
  [Thermistors_2R] -> Mux7/2
  [Thermistors_3L] -> Mux7/6
  [Thermistors_3R] -> Mux7/3
  Mux14/1 -> AbsoluteEncoders/1
  Mux12/1 -> IncrementalEncoders/1
  [ID_2L] -> Mux8/5
  [ID_IMU] -> Mux8/7
  [ID_1L] -> Mux8/4
  [ID_1R] -> Mux8/1
  [ID_2R] -> Mux8/2
  [ID_3R] -> Mux8/3
  [ID_3L] -> Mux8/6
  Mux8/1 -> MedullaID/1
  [LegEncoderTimestamp_1R] -> Mux9/1
  [LegEncoderTimestamp_2R] -> Mux9/2
  [LegEncoderTimestamp_1L] -> Mux9/3
  [LegEncoderTimestamp_2L] -> Mux9/4
  [MotorEncoderTimestamp_1R] -> Mux9/5
  [MotorEncoderTimestamp_2R] -> Mux9/6
  [MotorEncoderTimestamp_1L] -> Mux9/7
  [MotorEncoderTimestamp_2L] -> Mux9/8
  [HipEncoderTimestamp_3R] -> Mux9/9
  [HipEncoderTimestamp_3L] -> Mux9/10
  Mux9/1 -> AbsoluteEncoderTimestamps/1
  Data Type Conversion141/1 -> [IncEncoders_Boom]
  Mux13/1 -> IncrementalEncoderTimestamps/1
  [IncEncoderTimestamp_3R] -> Mux13/5
  [IncEncoderTimestamp_1R] -> Mux13/1
  [IncEncoderTimestamp_1L] -> Mux13/3
  [IncEncoderTimestamp_2L] -> Mux13/4
  [IncEncoderTimestamp_2R] -> Mux13/2
  [IncEncoderTimestamp_3L] -> Mux13/6
  Mux15/1 -> KneeForce/1
  [KneeForce_1R] -> Mux15/1
  [KneeForce_2R] -> Mux15/2
  [KneeForce_1L] -> Mux15/3
  [KneeForce_2L] -> Mux15/4
  IMU_Medulla/3(Accel) -> MicrostrainAcceleration/1
  IMU_Medulla/2(AngularRate) -> MicrostrainAngularRate/1
  Ground/1 -> Make3x1/1
  Make3x1/1 -> Data Type Conversion141/1
  [IncEncoders_Boom] -> Mux12/7
  Data Type Conversion16/1 -> [ID_IMU]
  Data Type Conversion17/1 -> [State_IMU]
  Data Type Conversion18/1 -> [Counter_IMU]
  Data Type Conversion19/1 -> [ErrorFlags_IMU]

== system StandaloneDAQv07_R2014a/EtherCATNetwork/IMUFilters ==
  q : Inport  Partition=on  PartitionDimension=1  PartitionWidth=1
  q_limits : Inport  Port=2  Partition=on  PartitionDimension=1  PartitionWidth=1
  Threshold : Inport  Port=3  Partition=off
  Reset : Inport  Port=4  Partition=off
  IMURate : Inport  Port=5  Partition=on  PartitionDimension=1  PartitionWidth=1
  UseIMURate : Inport  Port=6  Partition=off
  CheckAndFilterIMU : Subsystem
  For Each : ForEach  DisableCoverage=on  IndexMode=One-based
  q_clean : Outport  ConcatenationDimension=1
  dq_clean : Outport  Port=2  ConcatenationDimension=1
  ErrorCount : Outport  Port=3  ConcatenationDimension=1
  wires:
  UseIMURate/1 -> CheckAndFilterIMU/6(UseIMURate)
  IMURate/1 -> CheckAndFilterIMU/5(IMURate)
  q/1 -> CheckAndFilterIMU/1(q_daq)
  Threshold/1 -> CheckAndFilterIMU/3(Threshold)
  CheckAndFilterIMU/1(q_clean) -> q_clean/1
  CheckAndFilterIMU/3(ErrorCount) -> ErrorCount/1
  q_limits/1 -> CheckAndFilterIMU/2(q_limits)
  CheckAndFilterIMU/2(dq_clean) -> dq_clean/1
  Reset/1 -> CheckAndFilterIMU/4(Reset)

== system StandaloneDAQv07_R2014a/EtherCATNetwork/Reset ==
  note: EtherCATStatus is a vector of six elements:
      | [ErrVal MasterState DCErrVal MasterToNetworkClkDiff
      | DCInitState NetworkToSlaveClkDiff]
      | Here we just check that MasterState==8 (Operational state).
  ResetIn : Inport
  EtherCATStatus : Inport  Port=2
  Compare To Constant : simulink/Logic and Bit Operations/Compare To Constant  relop=<=  const=2.0  OutDataTypeStr=boolean
  Compare To Constant1 : simulink/Logic and Bit Operations/Compare To Constant  relop=~=  const=8  OutDataTypeStr=boolean
  Digital Clock : DigitalClock  SampleTime=0.0005
  Logical Operator : Logic  Operator=OR  Inputs=3  OutDataTypeStr=boolean
  Selector : Selector  IndexMode=Zero-based  InputPortWidth=6
  Reset : Outport
  wires:
  Selector/1 -> Compare To Constant1/1
  EtherCATStatus/1 -> Selector/1
  Compare To Constant1/1 -> Logical Operator/3
  Digital Clock/1 -> Compare To Constant/1
  Compare To Constant/1 -> Logical Operator/1
  ResetIn/1 -> Logical Operator/2
  Logical Operator/1 -> Reset/1

== system StandaloneDAQv07_R2014a/EtherCATNetwork/Subsystem ==
  Temp : Inport
  Counter : dspswit3/Counter  Direction=Up  CountEvent=Free running  CounterSize=User defined  MaxCount=29  InitialCount=0  Output=Count  HitValue=32  ResetInput=off  SamplesPerFrame=1  Ts=0.0005  CntDtype=uint8  HitDtype=Logical
  Discrete Filter : DiscreteFilter  Numerator=[1-0.99]  Denominator=[1 -0.99]  InitialStates=zeros(30,1)
  Index Vector : MultiPortSwitch  DataPortOrder=Zero-based contiguous  Inputs=1  zeroidx=on
  MxTemp : Outport
  wires:
  Temp/1 -> Discrete Filter/1
  Index Vector/1 -> MxTemp/1
  Discrete Filter/1 -> Index Vector/2
  Counter/1 -> Index Vector/1

== system StandaloneDAQv07_R2014a/SerialInterfaces/FTInterface ==
  Tare : Inport
  Reset : Inport  Port=2
  Enable : EnablePort
  ATI Serial NoInt : Subsystem  mask{irqnum=5, slot=[4 4]}
      mask prompts: irqnum "IRQ"; slot "PCI [bus slot]"
      mask TypeOptions irqnum: 5 | 9
      mask Callback irqnum: set_param([gcb '/Board Setup'], 'irqnum', num2str(get_param(gcb,'irqnum')));
      mask Display:
      | disp('IO503\nTPMC466\nSend Interrupt-Free\nReceive Interrup-Free')
      | 
      | port_label('input', 1, 'TX1')
      | port_label('input', 2, 'TX2')
      | 
      | port_label('output', 1, 'RX1')
      | port_label('output', 2, 'RX2')
  CalibrationSet : Constant
  Demux : Demux  Outputs=2
  Mux : Mux  Inputs=2
  Subsystem : Subsystem
  FTStatus : Outport  OutputWhenDisabled=reset  InitialOutput=zeros(2,1)
  FT : Outport  Port=2  OutputWhenDisabled=reset  InitialOutput=zeros(12,1)
  FTInterfaceStatus : Outport  Port=3  OutputWhenDisabled=reset  InitialOutput=zeros(2,1)
  FTSetupStatus : Outport  Port=4  OutputWhenDisabled=reset  InitialOutput=zeros(2,1)
  CalibrationSerial : Outport  Port=5  OutputWhenDisabled=reset  InitialOutput=zeros(2,1)
  wires:
  Subsystem/4(FTSetupStatus) -> FTSetupStatus/1
  Subsystem/3(FTInterfaceStatus) -> FTInterfaceStatus/1
  Subsystem/5(CalibrationSerial) -> CalibrationSerial/1
  CalibrationSet/1 -> Subsystem/1(CalibrationSet)
  Subsystem/2(FT) -> FT/1
  ATI Serial NoInt/2(RX2) -> Mux/2
  Subsystem/1(FTStatus) -> FTStatus/1
  Tare/1 -> Subsystem/2(Tare)
  Reset/1 -> Subsystem/3(Reset)
  Mux/1 -> Subsystem/4(SerialIn)
  Subsystem/6(SerialOut) -> Demux/1
  Demux/2 -> ATI Serial NoInt/2(TX2)
  Demux/1 -> ATI Serial NoInt/1(TX1)
  ATI Serial NoInt/1(RX1) -> Mux/1

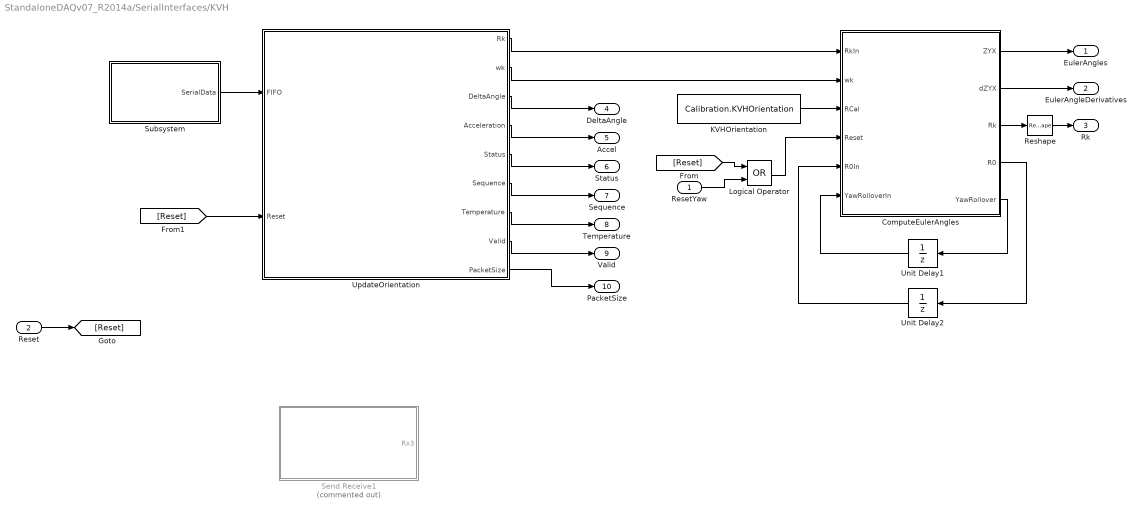
== system StandaloneDAQv07_R2014a/SerialInterfaces/KVH ==
  ResetYaw : Inport
  Reset : Inport  Port=2
  ComputeEulerAngles : MATLAB Function  TreatAsAtomicUnit=on
  KVHOrientation : Constant  Value=Calibration.KVHOrientation
  Logical Operator : Logic  Operator=OR  OutDataTypeStr=boolean
  Reshape : Reshape
  Send Receive1 : Subsystem  Commented=on  InitFcn=m_XR17D15x(3);  mask(sendreceive_IO503){slot=[4 5], irqnum=9}
      mask prompts: slot "PCI slot (-1: autosearch):"; irqnum "IRQ number:"
      mask help:
      | Speedgoat driver block
      | IO503 - Send Receive
      mask Help: web(fullfile(speedgoatroot,'sg_help','serial','dialog_fields_send_rec_io503.htm'),'-helpbrowser');
      mask Display:
      | disp('Speedgoat\nIO503\n422 Receive\nNo Interrupts');
      | 
      | port_label( 'output', 1, 'Rx3' );
  Subsystem : Subsystem  mask{irqnum=9, slot=[4 5]}
      mask prompts: irqnum "IRQ"; slot "PCI [bus slot]"
      mask TypeOptions irqnum: 5 | 9
      mask Callback irqnum: set_param([gcb '/Board Setup'], 'irqnum', num2str(get_param(gcb,'irqnum')));
      mask Display:
      | disp('Speedgoat\nIO503\nRS422 Receive\nInterrupt-free');
      | port_label( 'output', 1, 'RX3' );
  Unit Delay1 : UnitDelay  InitialCondition=[0; 0]  SampleTime=-1
  Unit Delay2 : UnitDelay  InitialCondition=zeros(3,3)  SampleTime=-1
  UpdateOrientation : Subsystem
  EulerAngles : Outport
  EulerAngleDerivatives : Outport  Port=2
  Rk : Outport  Port=3
  DeltaAngle : Outport  Port=4
  Accel : Outport  Port=5
  Status : Outport  Port=6
  Sequence : Outport  Port=7
  Temperature : Outport  Port=8
  Valid : Outport  Port=9
  PacketSize : Outport  Port=10
  wires:
  [Reset] -> UpdateOrientation/2(Reset)
  UpdateOrientation/5(Status) -> Status/1
  UpdateOrientation/7(Temperature) -> Temperature/1
  UpdateOrientation/4(Acceleration) -> Accel/1
  UpdateOrientation/3(DeltaAngle) -> DeltaAngle/1
  UpdateOrientation/8(Valid) -> Valid/1
  UpdateOrientation/6(Sequence) -> Sequence/1
  Reset/1 -> [Reset]
  KVHOrientation/1 -> ComputeEulerAngles/3(RCal)
  Unit Delay2/1 -> ComputeEulerAngles/5(R0In)
  ComputeEulerAngles/1(ZYX) -> EulerAngles/1
  ComputeEulerAngles/4(R0) -> Unit Delay2/1
  ComputeEulerAngles/3(Rk) -> Reshape/1
  [Reset] -> Logical Operator/1
  Reshape/1 -> Rk/1
  UpdateOrientation/1(Rk) -> ComputeEulerAngles/1(RkIn)
  UpdateOrientation/2(wk) -> ComputeEulerAngles/2(wk)
  ComputeEulerAngles/2(dZYX) -> EulerAngleDerivatives/1
  ComputeEulerAngles/5(YawRollover) -> Unit Delay1/1
  Unit Delay1/1 -> ComputeEulerAngles/6(YawRolloverIn)
  ResetYaw/1 -> Logical Operator/2
  Logical Operator/1 -> ComputeEulerAngles/4(Reset)
  Subsystem/1(SerialData) -> UpdateOrientation/1(FIFO)
  UpdateOrientation/9(PacketSize) -> PacketSize/1

== system StandaloneDAQv07_R2014a/EtherCATNetwork/EncoderFilters/CheckAndFilterEncoder ==
  q_daq : Inport
  q_limits : Inport  Port=2
  Threshold : Inport  Port=3
  Reset : Inport  Port=4
  Counter : Inport  Port=5
  AnomalyDetection : Stateflow chart  TreatAsAtomicUnit=on  SystemSampleTime=EncoderFiltSys.dt
  Constant : Constant  Value=EncoderFiltSys.dt
  Discrete State-Space : DiscreteStateSpace  A=EncoderFiltSys.A  B=EncoderFiltSys.B  C=EncoderFiltSys.C  D=EncoderFiltSys.D  X0=EncoderFiltSys.x0  SampleTime=EncoderFiltSys.dt
  Unit Delay : UnitDelay  SampleTime=EncoderFiltSys.dt
  q_clean : Outport
  dq_clean : Outport  Port=2
  ErrorCount : Outport  Port=3
  wires:
  Counter/1 -> AnomalyDetection/3(Counter)
  Reset/1 -> AnomalyDetection/6(Reset)
  AnomalyDetection/2(ErrorCount) -> ErrorCount/1
  q_limits/1 -> AnomalyDetection/4(q_limits)
  Constant/1 -> AnomalyDetection/7(ANOMALY_DT)
  Unit Delay/1 -> AnomalyDetection/2(dq)
  Threshold/1 -> AnomalyDetection/5(Threshold)
  q_daq/1 -> AnomalyDetection/1(q)
  Discrete State-Space/1 -> Unit Delay/1, dq_clean/1
  AnomalyDetection/1(q_clean) -> q_clean/1, Discrete State-Space/1
